simulink model "lyskawaLab8_si_rs"  (R2023b)
settings: Solver=VariableStepAuto  StartTime=startTime  StopTime=stopTime  MaxStep=maxStepSize  RelTol=1e-3
values from neighbouring files (symbols this model uses):
  dfwe1 = 0    [lyskawaLab8.m]
  dfwe2 = 0.1*fwe2max    [lyskawaLab8.m]
  fwe1_0 = 0.2*fwe1max    [lyskawaLab8.m]
  fwe2_0 = arrayfwe2_0(i)    [lyskawaLab8.m]
  h_0 = [h1_0, h2_0]    [lyskawaLab8.m]
  M1 = [-a1/A1, a1/A1;a1/A2, -a1/A2-a2/A2]    [lyskawaLab8.m]
  M2 = [1/A1, 0;0, 1/A2]    [lyskawaLab8.m]
  M3 = [1, 0;0, 1]    [lyskawaLab8.m]
  M4 = [0, 0;0, 0]    [lyskawaLab8.m]
  t0 = 5    [lyskawaLab8.m]
settings Model: Creator=aleklyskawa  LastModifiedBy=aleklyskawa

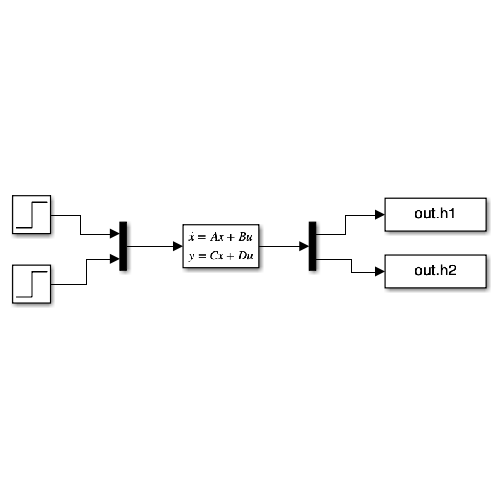
[thumbnail: Simulink's stored preview of the top-level diagram]
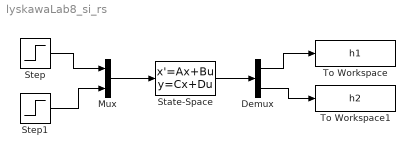
== system lyskawaLab8_si_rs ==
  Demux : Demux  Outputs=2
  Mux : Mux  Inputs=2
  State-Space : StateSpace  A=M1  B=M2  C=M3  D=M4  InitialCondition=h_0
  Step : Step  Time=t0  Before=fwe1_0  After=fwe1_0 + dfwe1  SampleTime=0
  Step1 : Step  Time=t0  Before=fwe2_0  After=fwe2_0 + dfwe2  SampleTime=0
  To Workspace : ToWorkspace  VariableName=h1  SampleTime=-1
  To Workspace1 : ToWorkspace  VariableName=h2  SampleTime=-1
  wires:
  Mux/1 -> State-Space/1
  Step1/1 -> Mux/2
  Step/1 -> Mux/1
  Demux/1 -> To Workspace/1
  Demux/2 -> To Workspace1/1
  State-Space/1 -> Demux/1
